simulink model "Open_scen_lucie_test_cs"  (R2019a)
settings: Solver=ode5  StartTime=0.0  StopTime=60  FixedStep=1/60  RelTol=1e-3
PreLoadFcn:
  | mbxruntime.callbacks.PreLoadFcn(bdroot);
PostLoadFcn:
  | mbxruntime.callbacks.PostLoadFcn(bdroot);
InitFcn:
  | mbxruntime.callbacks.InitFcn(bdroot);
StartFcn:
  | mbxruntime.callbacks.StartFcn(bdroot);
StopFcn:
  | mbxruntime.callbacks.StopFcn(bdroot);
model workspace: external: MAT-File .\Open_scen_lucie_test_cs_hws.mat (data not in the file)
undefined symbols (not defined in the file or in its folder): DiscIntNeverNeededParam, FovAzimuth, FovAzimuthDefined, FovElevation, FovElevationDefined, InitImageOutputDir, LocationX, LocationXDefined, LocationY, LocationYDefined, LocationZ, LocationZDefined, mbxruntime, Open_scen_lucie_test_cs_05b3fdca6ec99adc, Open_scen_lucie_test_cs_2d1bc0fbf6141b87, Open_scen_lucie_test_cs_453760b7ad36561d, Open_scen_lucie_test_cs_54de7300b247ce0d, Open_scen_lucie_test_cs_6819f386244a4b71, Open_scen_lucie_test_cs_685351e056f1bd0b, Open_scen_lucie_test_cs_6cd7f038842b0b77, Open_scen_lucie_test_cs_7a35ff65ce771bf6, Open_scen_lucie_test_cs_7ca083c9065fb1a1, Open_scen_lucie_test_cs_8bffacb258fa391b, Open_scen_lucie_test_cs_90e3bd399387ee5e, Open_scen_lucie_test_cs_a1176fb0c2e52fd1, Open_scen_lucie_test_cs_bb93306955583605, Open_scen_lucie_test_cs_c100ca66a180e443, Open_scen_lucie_test_cs_c1ddb1ec4c47a5f8, Open_scen_lucie_test_cs_ee3cfcef3d4d50fa, Open_scen_lucie_test_cs_f0142b471b498fb5, Open_scen_lucie_test_cs_fad1968c5de81336, OrientationPitch, OrientationPitchDefined, OrientationRoll, OrientationRollDefined, OrientationYaw, OrientationYawDefined, tabledata
libraries: adeye_lib x15, PreScanSimulinkLibrary x6, PreScanUsefulBlocks x1, simulink x1
(part 7 of 8)

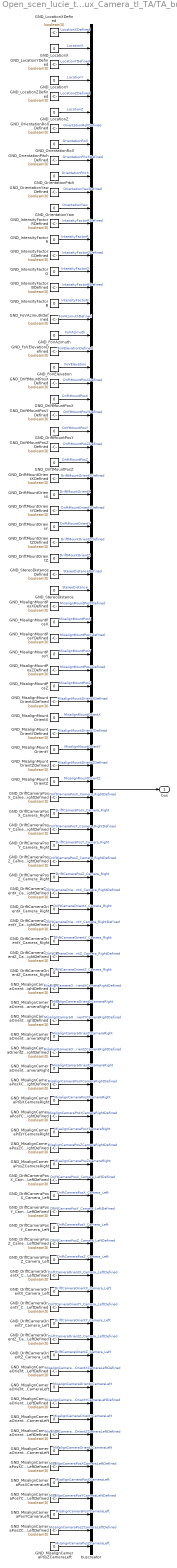
== system Open_scen_lucie_test_cs/BMW_X5_SUV_1/Mux_Camera_tl_TA/TA_bus ==
  GND_DriftCameraOrientX_Camera_Left : Constant  Value=0
  GND_DriftCameraOrientX_Camera_LeftDefined : Constant  Value=boolean(0)
  GND_DriftCameraOrientX_Camera_Right : Constant  Value=0
  GND_DriftCameraOrientX_Camera_RightDefined : Constant  Value=boolean(0)
  GND_DriftCameraOrientY_Camera_Left : Constant  Value=0
  GND_DriftCameraOrientY_Camera_LeftDefined : Constant  Value=boolean(0)
  GND_DriftCameraOrientY_Camera_Right : Constant  Value=0
  GND_DriftCameraOrientY_Camera_RightDefined : Constant  Value=boolean(0)
  GND_DriftCameraOrientZ_Camera_Left : Constant  Value=0
  GND_DriftCameraOrientZ_Camera_LeftDefined : Constant  Value=boolean(0)
  GND_DriftCameraOrientZ_Camera_Right : Constant  Value=0
  GND_DriftCameraOrientZ_Camera_RightDefined : Constant  Value=boolean(0)
  GND_DriftCameraPosX_Camera_Left : Constant  Value=0
  GND_DriftCameraPosX_Camera_LeftDefined : Constant  Value=boolean(0)
  GND_DriftCameraPosX_Camera_Right : Constant  Value=0
  GND_DriftCameraPosX_Camera_RightDefined : Constant  Value=boolean(0)
  GND_DriftCameraPosY_Camera_Left : Constant  Value=0
  GND_DriftCameraPosY_Camera_LeftDefined : Constant  Value=boolean(0)
  GND_DriftCameraPosY_Camera_Right : Constant  Value=0
  GND_DriftCameraPosY_Camera_RightDefined : Constant  Value=boolean(0)
  GND_DriftCameraPosZ_Camera_Left : Constant  Value=0
  GND_DriftCameraPosZ_Camera_LeftDefined : Constant  Value=boolean(0)
  GND_DriftCameraPosZ_Camera_Right : Constant  Value=0
  GND_DriftCameraPosZ_Camera_RightDefined : Constant  Value=boolean(0)
  GND_DriftMountOrientX : Constant  Value=0
  GND_DriftMountOrientXDefined : Constant  Value=boolean(0)
  GND_DriftMountOrientY : Constant  Value=0
  GND_DriftMountOrientYDefined : Constant  Value=boolean(0)
  GND_DriftMountOrientZ : Constant  Value=0
  GND_DriftMountOrientZDefined : Constant  Value=boolean(0)
  GND_DriftMountPosX : Constant  Value=0
  GND_DriftMountPosXDefined : Constant  Value=boolean(0)
  GND_DriftMountPosY : Constant  Value=0
  GND_DriftMountPosYDefined : Constant  Value=boolean(0)
  GND_DriftMountPosZ : Constant  Value=0
  GND_DriftMountPosZDefined : Constant  Value=boolean(0)
  GND_FoVAzimuth : Constant  Value=0
  GND_FoVAzimuthDefined : Constant  Value=boolean(0)
  GND_FoVElevation : Constant  Value=0
  GND_FoVElevationDefined : Constant  Value=boolean(0)
  GND_IntensityFactorB : Constant  Value=0
  GND_IntensityFactorBDefined : Constant  Value=boolean(0)
  GND_IntensityFactorG : Constant  Value=0
  GND_IntensityFactorGDefined : Constant  Value=boolean(0)
  GND_IntensityFactorR : Constant  Value=0
  GND_IntensityFactorRDefined : Constant  Value=boolean(0)
  GND_LocationX : Constant  Value=0
  GND_LocationXDefined : Constant  Value=boolean(0)
  GND_LocationY : Constant  Value=0
  GND_LocationYDefined : Constant  Value=boolean(0)
  GND_LocationZ : Constant  Value=0
  GND_LocationZDefined : Constant  Value=boolean(0)
  GND_MisalignCameraOrientXCameraLeft : Constant  Value=0
  GND_MisalignCameraOrientXCameraLeftDefined : Constant  Value=boolean(0)
  GND_MisalignCameraOrientXCameraRight : Constant  Value=0
  GND_MisalignCameraOrientXCameraRightDefined : Constant  Value=boolean(0)
  GND_MisalignCameraOrientYCameraLeft : Constant  Value=0
  GND_MisalignCameraOrientYCameraLeftDefined : Constant  Value=boolean(0)
  GND_MisalignCameraOrientYCameraRight : Constant  Value=0
  GND_MisalignCameraOrientYCameraRightDefined : Constant  Value=boolean(0)
  GND_MisalignCameraOrientZCameraLeft : Constant  Value=0
  GND_MisalignCameraOrientZCameraLeftDefined : Constant  Value=boolean(0)
  GND_MisalignCameraOrientZCameraRight : Constant  Value=0
  GND_MisalignCameraOrientZCameraRightDefined : Constant  Value=boolean(0)
  GND_MisalignCameraPosXCameraLeft : Constant  Value=0
  GND_MisalignCameraPosXCameraLeftDefined : Constant  Value=boolean(0)
  GND_MisalignCameraPosXCameraRight : Constant  Value=0
  GND_MisalignCameraPosXCameraRightDefined : Constant  Value=boolean(0)
  GND_MisalignCameraPosYCameraLeft : Constant  Value=0
  GND_MisalignCameraPosYCameraLeftDefined : Constant  Value=boolean(0)
  GND_MisalignCameraPosYCameraRight : Constant  Value=0
  GND_MisalignCameraPosYCameraRightDefined : Constant  Value=boolean(0)
  GND_MisalignCameraPosZCameraLeft : Constant  Value=0
  GND_MisalignCameraPosZCameraLeftDefined : Constant  Value=boolean(0)
  GND_MisalignCameraPosZCameraRight : Constant  Value=0
  GND_MisalignCameraPosZCameraRightDefined : Constant  Value=boolean(0)
  GND_MisalignMountOrientX : Constant  Value=0
  GND_MisalignMountOrientXDefined : Constant  Value=boolean(0)
  GND_MisalignMountOrientY : Constant  Value=0
  GND_MisalignMountOrientYDefined : Constant  Value=boolean(0)
  GND_MisalignMountOrientZ : Constant  Value=0
  GND_MisalignMountOrientZDefined : Constant  Value=boolean(0)
  GND_MisalignMountPosX : Constant  Value=0
  GND_MisalignMountPosXDefined : Constant  Value=boolean(0)
  GND_MisalignMountPosY : Constant  Value=0
  GND_MisalignMountPosYDefined : Constant  Value=boolean(0)
  GND_MisalignMountPosZ : Constant  Value=0
  GND_MisalignMountPosZDefined : Constant  Value=boolean(0)
  GND_OrientationPitch : Constant  Value=0
  GND_OrientationPitchDefined : Constant  Value=boolean(0)
  GND_OrientationRoll : Constant  Value=0
  GND_OrientationRollDefined : Constant  Value=boolean(0)
  GND_OrientationYaw : Constant  Value=0
  GND_OrientationYawDefined : Constant  Value=boolean(0)
  GND_StereoDistance : Constant  Value=0
  GND_StereoDistanceDefined : Constant  Value=boolean(0)
  buscreator : BusCreator  Inputs=96  OutDataTypeStr=Bus: PRESCAN_CAMERASENSOR_TA  NonVirtualBus=on
  bus : Outport  OutDataTypeStr=Bus: PRESCAN_CAMERASENSOR_TA
  wires:
  GND_LocationXDefined/1 -> buscreator/1  "LocationXDefined"
  GND_LocationX/1 -> buscreator/2  "LocationX"
  GND_LocationYDefined/1 -> buscreator/3  "LocationYDefined"
  GND_LocationY/1 -> buscreator/4  "LocationY"
  GND_LocationZDefined/1 -> buscreator/5  "LocationZDefined"
  GND_LocationZ/1 -> buscreator/6  "LocationZ"
  GND_OrientationRollDefined/1 -> buscreator/7  "OrientationRollDefined"
  GND_OrientationRoll/1 -> buscreator/8  "OrientationRoll"
  GND_OrientationPitchDefined/1 -> buscreator/9  "OrientationPitchDefined"
  GND_OrientationPitch/1 -> buscreator/10  "OrientationPitch"
  GND_OrientationYawDefined/1 -> buscreator/11  "OrientationYawDefined"
  GND_OrientationYaw/1 -> buscreator/12  "OrientationYaw"
  GND_IntensityFactorRDefined/1 -> buscreator/13  "IntensityFactorRDefined"
  GND_IntensityFactorR/1 -> buscreator/14  "IntensityFactorR"
  GND_IntensityFactorGDefined/1 -> buscreator/15  "IntensityFactorGDefined"
  GND_IntensityFactorG/1 -> buscreator/16  "IntensityFactorG"
  GND_IntensityFactorBDefined/1 -> buscreator/17  "IntensityFactorBDefined"
  GND_IntensityFactorB/1 -> buscreator/18  "IntensityFactorB"
  GND_FoVAzimuthDefined/1 -> buscreator/19  "FoVAzimuthDefined"
  GND_FoVAzimuth/1 -> buscreator/20  "FoVAzimuth"
  GND_FoVElevationDefined/1 -> buscreator/21  "FoVElevationDefined"
  GND_FoVElevation/1 -> buscreator/22  "FoVElevation"
  GND_DriftMountPosXDefined/1 -> buscreator/23  "DriftMountPosXDefined"
  GND_DriftMountPosX/1 -> buscreator/24  "DriftMountPosX"
  GND_DriftMountPosYDefined/1 -> buscreator/25  "DriftMountPosYDefined"
  GND_DriftMountPosY/1 -> buscreator/26  "DriftMountPosY"
  GND_DriftMountPosZDefined/1 -> buscreator/27  "DriftMountPosZDefined"
  GND_DriftMountPosZ/1 -> buscreator/28  "DriftMountPosZ"
  GND_DriftMountOrientXDefined/1 -> buscreator/29  "DriftMountOrientXDefined"
  GND_DriftMountOrientX/1 -> buscreator/30  "DriftMountOrientX"
  GND_DriftMountOrientYDefined/1 -> buscreator/31  "DriftMountOrientYDefined"
  GND_DriftMountOrientY/1 -> buscreator/32  "DriftMountOrientY"
  GND_DriftMountOrientZDefined/1 -> buscreator/33  "DriftMountOrientZDefined"
  GND_DriftMountOrientZ/1 -> buscreator/34  "DriftMountOrientZ"
  GND_StereoDistanceDefined/1 -> buscreator/35  "StereoDistanceDefined"
  GND_StereoDistance/1 -> buscreator/36  "StereoDistance"
  GND_MisalignMountPosXDefined/1 -> buscreator/37  "MisalignMountPosXDefined"
  GND_MisalignMountPosX/1 -> buscreator/38  "MisalignMountPosX"
  GND_MisalignMountPosYDefined/1 -> buscreator/39  "MisalignMountPosYDefined"
  GND_MisalignMountPosY/1 -> buscreator/40  "MisalignMountPosY"
  GND_MisalignMountPosZDefined/1 -> buscreator/41  "MisalignMountPosZDefined"
  GND_MisalignMountPosZ/1 -> buscreator/42  "MisalignMountPosZ"
  GND_MisalignMountOrientXDefined/1 -> buscreator/43  "MisalignMountOrientXDefined"
  GND_MisalignMountOrientX/1 -> buscreator/44  "MisalignMountOrientX"
  GND_MisalignMountOrientYDefined/1 -> buscreator/45  "MisalignMountOrientYDefined"
  GND_MisalignMountOrientY/1 -> buscreator/46  "MisalignMountOrientY"
  GND_MisalignMountOrientZDefined/1 -> buscreator/47  "MisalignMountOrientZDefined"
  GND_MisalignMountOrientZ/1 -> buscreator/48  "MisalignMountOrientZ"
  GND_DriftCameraPosX_Camera_RightDefined/1 -> buscreator/49  "DriftCameraPosX_Camera_RightDefined"
  GND_DriftCameraPosX_Camera_Right/1 -> buscreator/50  "DriftCameraPosX_Camera_Right"
  GND_DriftCameraPosY_Camera_RightDefined/1 -> buscreator/51  "DriftCameraPosY_Camera_RightDefined"
  GND_DriftCameraPosY_Camera_Right/1 -> buscreator/52  "DriftCameraPosY_Camera_Right"
  GND_DriftCameraPosZ_Camera_RightDefined/1 -> buscreator/53  "DriftCameraPosZ_Camera_RightDefined"
  GND_DriftCameraPosZ_Camera_Right/1 -> buscreator/54  "DriftCameraPosZ_Camera_Right"
  GND_DriftCameraOrientX_Camera_RightDefined/1 -> buscreator/55  "DriftCameraOrientX_Camera_RightDefined"
  GND_DriftCameraOrientX_Camera_Right/1 -> buscreator/56  "DriftCameraOrientX_Camera_Right"
  GND_DriftCameraOrientY_Camera_RightDefined/1 -> buscreator/57  "DriftCameraOrientY_Camera_RightDefined"
  GND_DriftCameraOrientY_Camera_Right/1 -> buscreator/58  "DriftCameraOrientY_Camera_Right"
  GND_DriftCameraOrientZ_Camera_RightDefined/1 -> buscreator/59  "DriftCameraOrientZ_Camera_RightDefined"
  GND_DriftCameraOrientZ_Camera_Right/1 -> buscreator/60  "DriftCameraOrientZ_Camera_Right"
  GND_MisalignCameraOrientXCameraRightDefined/1 -> buscreator/61  "MisalignCameraOrientXCameraRightDefined"
  GND_MisalignCameraOrientXCameraRight/1 -> buscreator/62  "MisalignCameraOrientXCameraRight"
  GND_MisalignCameraOrientYCameraRightDefined/1 -> buscreator/63  "MisalignCameraOrientYCameraRightDefined"
  GND_MisalignCameraOrientYCameraRight/1 -> buscreator/64  "MisalignCameraOrientYCameraRight"
  GND_MisalignCameraOrientZCameraRightDefined/1 -> buscreator/65  "MisalignCameraOrientZCameraRightDefined"
  GND_MisalignCameraOrientZCameraRight/1 -> buscreator/66  "MisalignCameraOrientZCameraRight"
  GND_MisalignCameraPosXCameraRightDefined/1 -> buscreator/67  "MisalignCameraPosXCameraRightDefined"
  GND_MisalignCameraPosXCameraRight/1 -> buscreator/68  "MisalignCameraPosXCameraRight"
  GND_MisalignCameraPosYCameraRightDefined/1 -> buscreator/69  "MisalignCameraPosYCameraRightDefined"
  GND_MisalignCameraPosYCameraRight/1 -> buscreator/70  "MisalignCameraPosYCameraRight"
  GND_MisalignCameraPosZCameraRightDefined/1 -> buscreator/71  "MisalignCameraPosZCameraRightDefined"
  GND_MisalignCameraPosZCameraRight/1 -> buscreator/72  "MisalignCameraPosZCameraRight"
  GND_DriftCameraPosX_Camera_LeftDefined/1 -> buscreator/73  "DriftCameraPosX_Camera_LeftDefined"
  GND_DriftCameraPosX_Camera_Left/1 -> buscreator/74  "DriftCameraPosX_Camera_Left"
  GND_DriftCameraPosY_Camera_LeftDefined/1 -> buscreator/75  "DriftCameraPosY_Camera_LeftDefined"
  GND_DriftCameraPosY_Camera_Left/1 -> buscreator/76  "DriftCameraPosY_Camera_Left"
  GND_DriftCameraPosZ_Camera_LeftDefined/1 -> buscreator/77  "DriftCameraPosZ_Camera_LeftDefined"
  GND_DriftCameraPosZ_Camera_Left/1 -> buscreator/78  "DriftCameraPosZ_Camera_Left"
  GND_DriftCameraOrientX_Camera_LeftDefined/1 -> buscreator/79  "DriftCameraOrientX_Camera_LeftDefined"
  GND_DriftCameraOrientX_Camera_Left/1 -> buscreator/80  "DriftCameraOrientX_Camera_Left"
  GND_DriftCameraOrientY_Camera_LeftDefined/1 -> buscreator/81  "DriftCameraOrientY_Camera_LeftDefined"
  GND_DriftCameraOrientY_Camera_Left/1 -> buscreator/82  "DriftCameraOrientY_Camera_Left"
  GND_DriftCameraOrientZ_Camera_LeftDefined/1 -> buscreator/83  "DriftCameraOrientZ_Camera_LeftDefined"
  GND_DriftCameraOrientZ_Camera_Left/1 -> buscreator/84  "DriftCameraOrientZ_Camera_Left"
  GND_MisalignCameraOrientXCameraLeftDefined/1 -> buscreator/85  "MisalignCameraOrientXCameraLeftDefined"
  GND_MisalignCameraOrientXCameraLeft/1 -> buscreator/86  "MisalignCameraOrientXCameraLeft"
  GND_MisalignCameraOrientYCameraLeftDefined/1 -> buscreator/87  "MisalignCameraOrientYCameraLeftDefined"
  GND_MisalignCameraOrientYCameraLeft/1 -> buscreator/88  "MisalignCameraOrientYCameraLeft"
  GND_MisalignCameraOrientZCameraLeftDefined/1 -> buscreator/89  "MisalignCameraOrientZCameraLeftDefined"
  GND_MisalignCameraOrientZCameraLeft/1 -> buscreator/90  "MisalignCameraOrientZCameraLeft"
  GND_MisalignCameraPosXCameraLeftDefined/1 -> buscreator/91  "MisalignCameraPosXCameraLeftDefined"
  GND_MisalignCameraPosXCameraLeft/1 -> buscreator/92  "MisalignCameraPosXCameraLeft"
  GND_MisalignCameraPosYCameraLeftDefined/1 -> buscreator/93  "MisalignCameraPosYCameraLeftDefined"
  GND_MisalignCameraPosYCameraLeft/1 -> buscreator/94  "MisalignCameraPosYCameraLeft"
  GND_MisalignCameraPosZCameraLeftDefined/1 -> buscreator/95  "MisalignCameraPosZCameraLeftDefined"
  GND_MisalignCameraPosZCameraLeft/1 -> buscreator/96  "MisalignCameraPosZCameraLeft"
  buscreator/1 -> bus/1

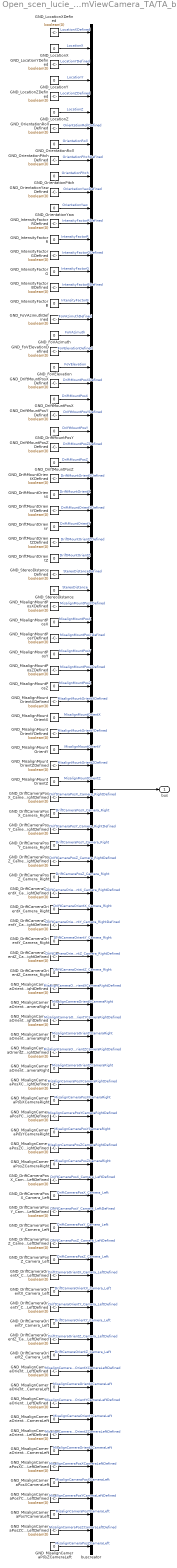
== system Open_scen_lucie_test_cs/BMW_X5_SUV_1/Mux_HumViewCamera_TA/TA_bus ==
  GND_DriftCameraOrientX_Camera_Left : Constant  Value=0
  GND_DriftCameraOrientX_Camera_LeftDefined : Constant  Value=boolean(0)
  GND_DriftCameraOrientX_Camera_Right : Constant  Value=0
  GND_DriftCameraOrientX_Camera_RightDefined : Constant  Value=boolean(0)
  GND_DriftCameraOrientY_Camera_Left : Constant  Value=0
  GND_DriftCameraOrientY_Camera_LeftDefined : Constant  Value=boolean(0)
  GND_DriftCameraOrientY_Camera_Right : Constant  Value=0
  GND_DriftCameraOrientY_Camera_RightDefined : Constant  Value=boolean(0)
  GND_DriftCameraOrientZ_Camera_Left : Constant  Value=0
  GND_DriftCameraOrientZ_Camera_LeftDefined : Constant  Value=boolean(0)
  GND_DriftCameraOrientZ_Camera_Right : Constant  Value=0
  GND_DriftCameraOrientZ_Camera_RightDefined : Constant  Value=boolean(0)
  GND_DriftCameraPosX_Camera_Left : Constant  Value=0
  GND_DriftCameraPosX_Camera_LeftDefined : Constant  Value=boolean(0)
  GND_DriftCameraPosX_Camera_Right : Constant  Value=0
  GND_DriftCameraPosX_Camera_RightDefined : Constant  Value=boolean(0)
  GND_DriftCameraPosY_Camera_Left : Constant  Value=0
  GND_DriftCameraPosY_Camera_LeftDefined : Constant  Value=boolean(0)
  GND_DriftCameraPosY_Camera_Right : Constant  Value=0
  GND_DriftCameraPosY_Camera_RightDefined : Constant  Value=boolean(0)
  GND_DriftCameraPosZ_Camera_Left : Constant  Value=0
  GND_DriftCameraPosZ_Camera_LeftDefined : Constant  Value=boolean(0)
  GND_DriftCameraPosZ_Camera_Right : Constant  Value=0
  GND_DriftCameraPosZ_Camera_RightDefined : Constant  Value=boolean(0)
  GND_DriftMountOrientX : Constant  Value=0
  GND_DriftMountOrientXDefined : Constant  Value=boolean(0)
  GND_DriftMountOrientY : Constant  Value=0
  GND_DriftMountOrientYDefined : Constant  Value=boolean(0)
  GND_DriftMountOrientZ : Constant  Value=0
  GND_DriftMountOrientZDefined : Constant  Value=boolean(0)
  GND_DriftMountPosX : Constant  Value=0
  GND_DriftMountPosXDefined : Constant  Value=boolean(0)
  GND_DriftMountPosY : Constant  Value=0
  GND_DriftMountPosYDefined : Constant  Value=boolean(0)
  GND_DriftMountPosZ : Constant  Value=0
  GND_DriftMountPosZDefined : Constant  Value=boolean(0)
  GND_FoVAzimuth : Constant  Value=0
  GND_FoVAzimuthDefined : Constant  Value=boolean(0)
  GND_FoVElevation : Constant  Value=0
  GND_FoVElevationDefined : Constant  Value=boolean(0)
  GND_IntensityFactorB : Constant  Value=0
  GND_IntensityFactorBDefined : Constant  Value=boolean(0)
  GND_IntensityFactorG : Constant  Value=0
  GND_IntensityFactorGDefined : Constant  Value=boolean(0)
  GND_IntensityFactorR : Constant  Value=0
  GND_IntensityFactorRDefined : Constant  Value=boolean(0)
  GND_LocationX : Constant  Value=0
  GND_LocationXDefined : Constant  Value=boolean(0)
  GND_LocationY : Constant  Value=0
  GND_LocationYDefined : Constant  Value=boolean(0)
  GND_LocationZ : Constant  Value=0
  GND_LocationZDefined : Constant  Value=boolean(0)
  GND_MisalignCameraOrientXCameraLeft : Constant  Value=0
  GND_MisalignCameraOrientXCameraLeftDefined : Constant  Value=boolean(0)
  GND_MisalignCameraOrientXCameraRight : Constant  Value=0
  GND_MisalignCameraOrientXCameraRightDefined : Constant  Value=boolean(0)
  GND_MisalignCameraOrientYCameraLeft : Constant  Value=0
  GND_MisalignCameraOrientYCameraLeftDefined : Constant  Value=boolean(0)
  GND_MisalignCameraOrientYCameraRight : Constant  Value=0
  GND_MisalignCameraOrientYCameraRightDefined : Constant  Value=boolean(0)
  GND_MisalignCameraOrientZCameraLeft : Constant  Value=0
  GND_MisalignCameraOrientZCameraLeftDefined : Constant  Value=boolean(0)
  GND_MisalignCameraOrientZCameraRight : Constant  Value=0
  GND_MisalignCameraOrientZCameraRightDefined : Constant  Value=boolean(0)
  GND_MisalignCameraPosXCameraLeft : Constant  Value=0
  GND_MisalignCameraPosXCameraLeftDefined : Constant  Value=boolean(0)
  GND_MisalignCameraPosXCameraRight : Constant  Value=0
  GND_MisalignCameraPosXCameraRightDefined : Constant  Value=boolean(0)
  GND_MisalignCameraPosYCameraLeft : Constant  Value=0
  GND_MisalignCameraPosYCameraLeftDefined : Constant  Value=boolean(0)
  GND_MisalignCameraPosYCameraRight : Constant  Value=0
  GND_MisalignCameraPosYCameraRightDefined : Constant  Value=boolean(0)
  GND_MisalignCameraPosZCameraLeft : Constant  Value=0
  GND_MisalignCameraPosZCameraLeftDefined : Constant  Value=boolean(0)
  GND_MisalignCameraPosZCameraRight : Constant  Value=0
  GND_MisalignCameraPosZCameraRightDefined : Constant  Value=boolean(0)
  GND_MisalignMountOrientX : Constant  Value=0
  GND_MisalignMountOrientXDefined : Constant  Value=boolean(0)
  GND_MisalignMountOrientY : Constant  Value=0
  GND_MisalignMountOrientYDefined : Constant  Value=boolean(0)
  GND_MisalignMountOrientZ : Constant  Value=0
  GND_MisalignMountOrientZDefined : Constant  Value=boolean(0)
  GND_MisalignMountPosX : Constant  Value=0
  GND_MisalignMountPosXDefined : Constant  Value=boolean(0)
  GND_MisalignMountPosY : Constant  Value=0
  GND_MisalignMountPosYDefined : Constant  Value=boolean(0)
  GND_MisalignMountPosZ : Constant  Value=0
  GND_MisalignMountPosZDefined : Constant  Value=boolean(0)
  GND_OrientationPitch : Constant  Value=0
  GND_OrientationPitchDefined : Constant  Value=boolean(0)
  GND_OrientationRoll : Constant  Value=0
  GND_OrientationRollDefined : Constant  Value=boolean(0)
  GND_OrientationYaw : Constant  Value=0
  GND_OrientationYawDefined : Constant  Value=boolean(0)
  GND_StereoDistance : Constant  Value=0
  GND_StereoDistanceDefined : Constant  Value=boolean(0)
  buscreator : BusCreator  Inputs=96  OutDataTypeStr=Bus: PRESCAN_CAMERASENSOR_TA  NonVirtualBus=on
  bus : Outport  OutDataTypeStr=Bus: PRESCAN_CAMERASENSOR_TA
  wires:
  GND_LocationXDefined/1 -> buscreator/1  "LocationXDefined"
  GND_LocationX/1 -> buscreator/2  "LocationX"
  GND_LocationYDefined/1 -> buscreator/3  "LocationYDefined"
  GND_LocationY/1 -> buscreator/4  "LocationY"
  GND_LocationZDefined/1 -> buscreator/5  "LocationZDefined"
  GND_LocationZ/1 -> buscreator/6  "LocationZ"
  GND_OrientationRollDefined/1 -> buscreator/7  "OrientationRollDefined"
  GND_OrientationRoll/1 -> buscreator/8  "OrientationRoll"
  GND_OrientationPitchDefined/1 -> buscreator/9  "OrientationPitchDefined"
  GND_OrientationPitch/1 -> buscreator/10  "OrientationPitch"
  GND_OrientationYawDefined/1 -> buscreator/11  "OrientationYawDefined"
  GND_OrientationYaw/1 -> buscreator/12  "OrientationYaw"
  GND_IntensityFactorRDefined/1 -> buscreator/13  "IntensityFactorRDefined"
  GND_IntensityFactorR/1 -> buscreator/14  "IntensityFactorR"
  GND_IntensityFactorGDefined/1 -> buscreator/15  "IntensityFactorGDefined"
  GND_IntensityFactorG/1 -> buscreator/16  "IntensityFactorG"
  GND_IntensityFactorBDefined/1 -> buscreator/17  "IntensityFactorBDefined"
  GND_IntensityFactorB/1 -> buscreator/18  "IntensityFactorB"
  GND_FoVAzimuthDefined/1 -> buscreator/19  "FoVAzimuthDefined"
  GND_FoVAzimuth/1 -> buscreator/20  "FoVAzimuth"
  GND_FoVElevationDefined/1 -> buscreator/21  "FoVElevationDefined"
  GND_FoVElevation/1 -> buscreator/22  "FoVElevation"
  GND_DriftMountPosXDefined/1 -> buscreator/23  "DriftMountPosXDefined"
  GND_DriftMountPosX/1 -> buscreator/24  "DriftMountPosX"
  GND_DriftMountPosYDefined/1 -> buscreator/25  "DriftMountPosYDefined"
  GND_DriftMountPosY/1 -> buscreator/26  "DriftMountPosY"
  GND_DriftMountPosZDefined/1 -> buscreator/27  "DriftMountPosZDefined"
  GND_DriftMountPosZ/1 -> buscreator/28  "DriftMountPosZ"
  GND_DriftMountOrientXDefined/1 -> buscreator/29  "DriftMountOrientXDefined"
  GND_DriftMountOrientX/1 -> buscreator/30  "DriftMountOrientX"
  GND_DriftMountOrientYDefined/1 -> buscreator/31  "DriftMountOrientYDefined"
  GND_DriftMountOrientY/1 -> buscreator/32  "DriftMountOrientY"
  GND_DriftMountOrientZDefined/1 -> buscreator/33  "DriftMountOrientZDefined"
  GND_DriftMountOrientZ/1 -> buscreator/34  "DriftMountOrientZ"
  GND_StereoDistanceDefined/1 -> buscreator/35  "StereoDistanceDefined"
  GND_StereoDistance/1 -> buscreator/36  "StereoDistance"
  GND_MisalignMountPosXDefined/1 -> buscreator/37  "MisalignMountPosXDefined"
  GND_MisalignMountPosX/1 -> buscreator/38  "MisalignMountPosX"
  GND_MisalignMountPosYDefined/1 -> buscreator/39  "MisalignMountPosYDefined"
  GND_MisalignMountPosY/1 -> buscreator/40  "MisalignMountPosY"
  GND_MisalignMountPosZDefined/1 -> buscreator/41  "MisalignMountPosZDefined"
  GND_MisalignMountPosZ/1 -> buscreator/42  "MisalignMountPosZ"
  GND_MisalignMountOrientXDefined/1 -> buscreator/43  "MisalignMountOrientXDefined"
  GND_MisalignMountOrientX/1 -> buscreator/44  "MisalignMountOrientX"
  GND_MisalignMountOrientYDefined/1 -> buscreator/45  "MisalignMountOrientYDefined"
  GND_MisalignMountOrientY/1 -> buscreator/46  "MisalignMountOrientY"
  GND_MisalignMountOrientZDefined/1 -> buscreator/47  "MisalignMountOrientZDefined"
  GND_MisalignMountOrientZ/1 -> buscreator/48  "MisalignMountOrientZ"
  GND_DriftCameraPosX_Camera_RightDefined/1 -> buscreator/49  "DriftCameraPosX_Camera_RightDefined"
  GND_DriftCameraPosX_Camera_Right/1 -> buscreator/50  "DriftCameraPosX_Camera_Right"
  GND_DriftCameraPosY_Camera_RightDefined/1 -> buscreator/51  "DriftCameraPosY_Camera_RightDefined"
  GND_DriftCameraPosY_Camera_Right/1 -> buscreator/52  "DriftCameraPosY_Camera_Right"
  GND_DriftCameraPosZ_Camera_RightDefined/1 -> buscreator/53  "DriftCameraPosZ_Camera_RightDefined"
  GND_DriftCameraPosZ_Camera_Right/1 -> buscreator/54  "DriftCameraPosZ_Camera_Right"
  GND_DriftCameraOrientX_Camera_RightDefined/1 -> buscreator/55  "DriftCameraOrientX_Camera_RightDefined"
  GND_DriftCameraOrientX_Camera_Right/1 -> buscreator/56  "DriftCameraOrientX_Camera_Right"
  GND_DriftCameraOrientY_Camera_RightDefined/1 -> buscreator/57  "DriftCameraOrientY_Camera_RightDefined"
  GND_DriftCameraOrientY_Camera_Right/1 -> buscreator/58  "DriftCameraOrientY_Camera_Right"
  GND_DriftCameraOrientZ_Camera_RightDefined/1 -> buscreator/59  "DriftCameraOrientZ_Camera_RightDefined"
  GND_DriftCameraOrientZ_Camera_Right/1 -> buscreator/60  "DriftCameraOrientZ_Camera_Right"
  GND_MisalignCameraOrientXCameraRightDefined/1 -> buscreator/61  "MisalignCameraOrientXCameraRightDefined"
  GND_MisalignCameraOrientXCameraRight/1 -> buscreator/62  "MisalignCameraOrientXCameraRight"
  GND_MisalignCameraOrientYCameraRightDefined/1 -> buscreator/63  "MisalignCameraOrientYCameraRightDefined"
  GND_MisalignCameraOrientYCameraRight/1 -> buscreator/64  "MisalignCameraOrientYCameraRight"
  GND_MisalignCameraOrientZCameraRightDefined/1 -> buscreator/65  "MisalignCameraOrientZCameraRightDefined"
  GND_MisalignCameraOrientZCameraRight/1 -> buscreator/66  "MisalignCameraOrientZCameraRight"
  GND_MisalignCameraPosXCameraRightDefined/1 -> buscreator/67  "MisalignCameraPosXCameraRightDefined"
  GND_MisalignCameraPosXCameraRight/1 -> buscreator/68  "MisalignCameraPosXCameraRight"
  GND_MisalignCameraPosYCameraRightDefined/1 -> buscreator/69  "MisalignCameraPosYCameraRightDefined"
  GND_MisalignCameraPosYCameraRight/1 -> buscreator/70  "MisalignCameraPosYCameraRight"
  GND_MisalignCameraPosZCameraRightDefined/1 -> buscreator/71  "MisalignCameraPosZCameraRightDefined"
  GND_MisalignCameraPosZCameraRight/1 -> buscreator/72  "MisalignCameraPosZCameraRight"
  GND_DriftCameraPosX_Camera_LeftDefined/1 -> buscreator/73  "DriftCameraPosX_Camera_LeftDefined"
  GND_DriftCameraPosX_Camera_Left/1 -> buscreator/74  "DriftCameraPosX_Camera_Left"
  GND_DriftCameraPosY_Camera_LeftDefined/1 -> buscreator/75  "DriftCameraPosY_Camera_LeftDefined"
  GND_DriftCameraPosY_Camera_Left/1 -> buscreator/76  "DriftCameraPosY_Camera_Left"
  GND_DriftCameraPosZ_Camera_LeftDefined/1 -> buscreator/77  "DriftCameraPosZ_Camera_LeftDefined"
  GND_DriftCameraPosZ_Camera_Left/1 -> buscreator/78  "DriftCameraPosZ_Camera_Left"
  GND_DriftCameraOrientX_Camera_LeftDefined/1 -> buscreator/79  "DriftCameraOrientX_Camera_LeftDefined"
  GND_DriftCameraOrientX_Camera_Left/1 -> buscreator/80  "DriftCameraOrientX_Camera_Left"
  GND_DriftCameraOrientY_Camera_LeftDefined/1 -> buscreator/81  "DriftCameraOrientY_Camera_LeftDefined"
  GND_DriftCameraOrientY_Camera_Left/1 -> buscreator/82  "DriftCameraOrientY_Camera_Left"
  GND_DriftCameraOrientZ_Camera_LeftDefined/1 -> buscreator/83  "DriftCameraOrientZ_Camera_LeftDefined"
  GND_DriftCameraOrientZ_Camera_Left/1 -> buscreator/84  "DriftCameraOrientZ_Camera_Left"
  GND_MisalignCameraOrientXCameraLeftDefined/1 -> buscreator/85  "MisalignCameraOrientXCameraLeftDefined"
  GND_MisalignCameraOrientXCameraLeft/1 -> buscreator/86  "MisalignCameraOrientXCameraLeft"
  GND_MisalignCameraOrientYCameraLeftDefined/1 -> buscreator/87  "MisalignCameraOrientYCameraLeftDefined"
  GND_MisalignCameraOrientYCameraLeft/1 -> buscreator/88  "MisalignCameraOrientYCameraLeft"
  GND_MisalignCameraOrientZCameraLeftDefined/1 -> buscreator/89  "MisalignCameraOrientZCameraLeftDefined"
  GND_MisalignCameraOrientZCameraLeft/1 -> buscreator/90  "MisalignCameraOrientZCameraLeft"
  GND_MisalignCameraPosXCameraLeftDefined/1 -> buscreator/91  "MisalignCameraPosXCameraLeftDefined"
  GND_MisalignCameraPosXCameraLeft/1 -> buscreator/92  "MisalignCameraPosXCameraLeft"
  GND_MisalignCameraPosYCameraLeftDefined/1 -> buscreator/93  "MisalignCameraPosYCameraLeftDefined"
  GND_MisalignCameraPosYCameraLeft/1 -> buscreator/94  "MisalignCameraPosYCameraLeft"
  GND_MisalignCameraPosZCameraLeftDefined/1 -> buscreator/95  "MisalignCameraPosZCameraLeftDefined"
  GND_MisalignCameraPosZCameraLeft/1 -> buscreator/96  "MisalignCameraPosZCameraLeft"
  buscreator/1 -> bus/1

== system Open_scen_lucie_test_cs/BMW_X5_SUV_1/Mux_PointCloudSensor_1_TA/TA_bus ==
  GND_FarClippingDistance : Constant  Value=0
  GND_FarClippingDistanceDefined : Constant  Value=boolean(0)
  GND_FovAzimuth : Constant  Value=0
  GND_FovAzimuthDefined : Constant  Value=boolean(0)
  GND_FovElevation : Constant  Value=0
  GND_FovElevationDefined : Constant  Value=boolean(0)
  GND_LocationX : Constant  Value=0
  GND_LocationXDefined : Constant  Value=boolean(0)
  GND_LocationY : Constant  Value=0
  GND_LocationYDefined : Constant  Value=boolean(0)
  GND_LocationZ : Constant  Value=0
  GND_LocationZDefined : Constant  Value=boolean(0)
  GND_NearClippingDistance : Constant  Value=0
  GND_NearClippingDistanceDefined : Constant  Value=boolean(0)
  GND_OrientationPitch : Constant  Value=0
  GND_OrientationPitchDefined : Constant  Value=boolean(0)
  GND_OrientationRoll : Constant  Value=0
  GND_OrientationRollDefined : Constant  Value=boolean(0)
  GND_OrientationYaw : Constant  Value=0
  GND_OrientationYawDefined : Constant  Value=boolean(0)
  buscreator : BusCreator  Inputs=20  OutDataTypeStr=Bus: PRESCAN_PCS_TA_DATA  NonVirtualBus=on
  bus : Outport  OutDataTypeStr=Bus: PRESCAN_PCS_TA_DATA
  wires:
  GND_LocationXDefined/1 -> buscreator/1  "LocationXDefined"
  GND_LocationX/1 -> buscreator/2  "LocationX"
  GND_LocationYDefined/1 -> buscreator/3  "LocationYDefined"
  GND_LocationY/1 -> buscreator/4  "LocationY"
  GND_LocationZDefined/1 -> buscreator/5  "LocationZDefined"
  GND_LocationZ/1 -> buscreator/6  "LocationZ"
  GND_OrientationRollDefined/1 -> buscreator/7  "OrientationRollDefined"
  GND_OrientationRoll/1 -> buscreator/8  "OrientationRoll"
  GND_OrientationPitchDefined/1 -> buscreator/9  "OrientationPitchDefined"
  GND_OrientationPitch/1 -> buscreator/10  "OrientationPitch"
  GND_OrientationYawDefined/1 -> buscreator/11  "OrientationYawDefined"
  GND_OrientationYaw/1 -> buscreator/12  "OrientationYaw"
  GND_FovAzimuthDefined/1 -> buscreator/13  "FovAzimuthDefined"
  GND_FovAzimuth/1 -> buscreator/14  "FovAzimuth"
  GND_FovElevationDefined/1 -> buscreator/15  "FovElevationDefined"
  GND_FovElevation/1 -> buscreator/16  "FovElevation"
  GND_NearClippingDistanceDefined/1 -> buscreator/17  "NearClippingDistanceDefined"
  GND_NearClippingDistance/1 -> buscreator/18  "NearClippingDistance"
  GND_FarClippingDistanceDefined/1 -> buscreator/19  "FarClippingDistanceDefined"
  GND_FarClippingDistance/1 -> buscreator/20  "FarClippingDistance"
  buscreator/1 -> bus/1

== system Open_scen_lucie_test_cs/BMW_X5_SUV_1/Mux_PointCloudSensor_2_TA/TA_bus ==
  GND_FarClippingDistance : Constant  Value=0
  GND_FarClippingDistanceDefined : Constant  Value=boolean(0)
  GND_FovAzimuth : Constant  Value=0
  GND_FovAzimuthDefined : Constant  Value=boolean(0)
  GND_FovElevation : Constant  Value=0
  GND_FovElevationDefined : Constant  Value=boolean(0)
  GND_LocationX : Constant  Value=0
  GND_LocationXDefined : Constant  Value=boolean(0)
  GND_LocationY : Constant  Value=0
  GND_LocationYDefined : Constant  Value=boolean(0)
  GND_LocationZ : Constant  Value=0
  GND_LocationZDefined : Constant  Value=boolean(0)
  GND_NearClippingDistance : Constant  Value=0
  GND_NearClippingDistanceDefined : Constant  Value=boolean(0)
  GND_OrientationPitch : Constant  Value=0
  GND_OrientationPitchDefined : Constant  Value=boolean(0)
  GND_OrientationRoll : Constant  Value=0
  GND_OrientationRollDefined : Constant  Value=boolean(0)
  GND_OrientationYaw : Constant  Value=0
  GND_OrientationYawDefined : Constant  Value=boolean(0)
  buscreator : BusCreator  Inputs=20  OutDataTypeStr=Bus: PRESCAN_PCS_TA_DATA  NonVirtualBus=on
  bus : Outport  OutDataTypeStr=Bus: PRESCAN_PCS_TA_DATA
  wires:
  GND_LocationXDefined/1 -> buscreator/1  "LocationXDefined"
  GND_LocationX/1 -> buscreator/2  "LocationX"
  GND_LocationYDefined/1 -> buscreator/3  "LocationYDefined"
  GND_LocationY/1 -> buscreator/4  "LocationY"
  GND_LocationZDefined/1 -> buscreator/5  "LocationZDefined"
  GND_LocationZ/1 -> buscreator/6  "LocationZ"
  GND_OrientationRollDefined/1 -> buscreator/7  "OrientationRollDefined"
  GND_OrientationRoll/1 -> buscreator/8  "OrientationRoll"
  GND_OrientationPitchDefined/1 -> buscreator/9  "OrientationPitchDefined"
  GND_OrientationPitch/1 -> buscreator/10  "OrientationPitch"
  GND_OrientationYawDefined/1 -> buscreator/11  "OrientationYawDefined"
  GND_OrientationYaw/1 -> buscreator/12  "OrientationYaw"
  GND_FovAzimuthDefined/1 -> buscreator/13  "FovAzimuthDefined"
  GND_FovAzimuth/1 -> buscreator/14  "FovAzimuth"
  GND_FovElevationDefined/1 -> buscreator/15  "FovElevationDefined"
  GND_FovElevation/1 -> buscreator/16  "FovElevation"
  GND_NearClippingDistanceDefined/1 -> buscreator/17  "NearClippingDistanceDefined"
  GND_NearClippingDistance/1 -> buscreator/18  "NearClippingDistance"
  GND_FarClippingDistanceDefined/1 -> buscreator/19  "FarClippingDistanceDefined"
  GND_FarClippingDistance/1 -> buscreator/20  "FarClippingDistance"
  buscreator/1 -> bus/1

== system Open_scen_lucie_test_cs/BMW_X5_SUV_1/Mux_PointCloudSensor_3_TA/TA_bus ==
  GND_FarClippingDistance : Constant  Value=0
  GND_FarClippingDistanceDefined : Constant  Value=boolean(0)
  GND_FovAzimuth : Constant  Value=0
  GND_FovAzimuthDefined : Constant  Value=boolean(0)
  GND_FovElevation : Constant  Value=0
  GND_FovElevationDefined : Constant  Value=boolean(0)
  GND_LocationX : Constant  Value=0
  GND_LocationXDefined : Constant  Value=boolean(0)
  GND_LocationY : Constant  Value=0
  GND_LocationYDefined : Constant  Value=boolean(0)
  GND_LocationZ : Constant  Value=0
  GND_LocationZDefined : Constant  Value=boolean(0)
  GND_NearClippingDistance : Constant  Value=0
  GND_NearClippingDistanceDefined : Constant  Value=boolean(0)
  GND_OrientationPitch : Constant  Value=0
  GND_OrientationPitchDefined : Constant  Value=boolean(0)
  GND_OrientationRoll : Constant  Value=0
  GND_OrientationRollDefined : Constant  Value=boolean(0)
  GND_OrientationYaw : Constant  Value=0
  GND_OrientationYawDefined : Constant  Value=boolean(0)
  buscreator : BusCreator  Inputs=20  OutDataTypeStr=Bus: PRESCAN_PCS_TA_DATA  NonVirtualBus=on
  bus : Outport  OutDataTypeStr=Bus: PRESCAN_PCS_TA_DATA
  wires:
  GND_LocationXDefined/1 -> buscreator/1  "LocationXDefined"
  GND_LocationX/1 -> buscreator/2  "LocationX"
  GND_LocationYDefined/1 -> buscreator/3  "LocationYDefined"
  GND_LocationY/1 -> buscreator/4  "LocationY"
  GND_LocationZDefined/1 -> buscreator/5  "LocationZDefined"
  GND_LocationZ/1 -> buscreator/6  "LocationZ"
  GND_OrientationRollDefined/1 -> buscreator/7  "OrientationRollDefined"
  GND_OrientationRoll/1 -> buscreator/8  "OrientationRoll"
  GND_OrientationPitchDefined/1 -> buscreator/9  "OrientationPitchDefined"
  GND_OrientationPitch/1 -> buscreator/10  "OrientationPitch"
  GND_OrientationYawDefined/1 -> buscreator/11  "OrientationYawDefined"
  GND_OrientationYaw/1 -> buscreator/12  "OrientationYaw"
  GND_FovAzimuthDefined/1 -> buscreator/13  "FovAzimuthDefined"
  GND_FovAzimuth/1 -> buscreator/14  "FovAzimuth"
  GND_FovElevationDefined/1 -> buscreator/15  "FovElevationDefined"
  GND_FovElevation/1 -> buscreator/16  "FovElevation"
  GND_NearClippingDistanceDefined/1 -> buscreator/17  "NearClippingDistanceDefined"
  GND_NearClippingDistance/1 -> buscreator/18  "NearClippingDistance"
  GND_FarClippingDistanceDefined/1 -> buscreator/19  "FarClippingDistanceDefined"
  GND_FarClippingDistance/1 -> buscreator/20  "FarClippingDistance"
  buscreator/1 -> bus/1

== system Open_scen_lucie_test_cs/BMW_X5_SUV_1/Mux_PointCloudSensor_4_TA/TA_bus ==
  GND_FarClippingDistance : Constant  Value=0
  GND_FarClippingDistanceDefined : Constant  Value=boolean(0)
  GND_FovAzimuth : Constant  Value=0
  GND_FovAzimuthDefined : Constant  Value=boolean(0)
  GND_FovElevation : Constant  Value=0
  GND_FovElevationDefined : Constant  Value=boolean(0)
  GND_LocationX : Constant  Value=0
  GND_LocationXDefined : Constant  Value=boolean(0)
  GND_LocationY : Constant  Value=0
  GND_LocationYDefined : Constant  Value=boolean(0)
  GND_LocationZ : Constant  Value=0
  GND_LocationZDefined : Constant  Value=boolean(0)
  GND_NearClippingDistance : Constant  Value=0
  GND_NearClippingDistanceDefined : Constant  Value=boolean(0)
  GND_OrientationPitch : Constant  Value=0
  GND_OrientationPitchDefined : Constant  Value=boolean(0)
  GND_OrientationRoll : Constant  Value=0
  GND_OrientationRollDefined : Constant  Value=boolean(0)
  GND_OrientationYaw : Constant  Value=0
  GND_OrientationYawDefined : Constant  Value=boolean(0)
  buscreator : BusCreator  Inputs=20  OutDataTypeStr=Bus: PRESCAN_PCS_TA_DATA  NonVirtualBus=on
  bus : Outport  OutDataTypeStr=Bus: PRESCAN_PCS_TA_DATA
  wires:
  GND_LocationXDefined/1 -> buscreator/1  "LocationXDefined"
  GND_LocationX/1 -> buscreator/2  "LocationX"
  GND_LocationYDefined/1 -> buscreator/3  "LocationYDefined"
  GND_LocationY/1 -> buscreator/4  "LocationY"
  GND_LocationZDefined/1 -> buscreator/5  "LocationZDefined"
  GND_LocationZ/1 -> buscreator/6  "LocationZ"
  GND_OrientationRollDefined/1 -> buscreator/7  "OrientationRollDefined"
  GND_OrientationRoll/1 -> buscreator/8  "OrientationRoll"
  GND_OrientationPitchDefined/1 -> buscreator/9  "OrientationPitchDefined"
  GND_OrientationPitch/1 -> buscreator/10  "OrientationPitch"
  GND_OrientationYawDefined/1 -> buscreator/11  "OrientationYawDefined"
  GND_OrientationYaw/1 -> buscreator/12  "OrientationYaw"
  GND_FovAzimuthDefined/1 -> buscreator/13  "FovAzimuthDefined"
  GND_FovAzimuth/1 -> buscreator/14  "FovAzimuth"
  GND_FovElevationDefined/1 -> buscreator/15  "FovElevationDefined"
  GND_FovElevation/1 -> buscreator/16  "FovElevation"
  GND_NearClippingDistanceDefined/1 -> buscreator/17  "NearClippingDistanceDefined"
  GND_NearClippingDistance/1 -> buscreator/18  "NearClippingDistance"
  GND_FarClippingDistanceDefined/1 -> buscreator/19  "FarClippingDistanceDefined"
  GND_FarClippingDistance/1 -> buscreator/20  "FarClippingDistance"
  buscreator/1 -> bus/1

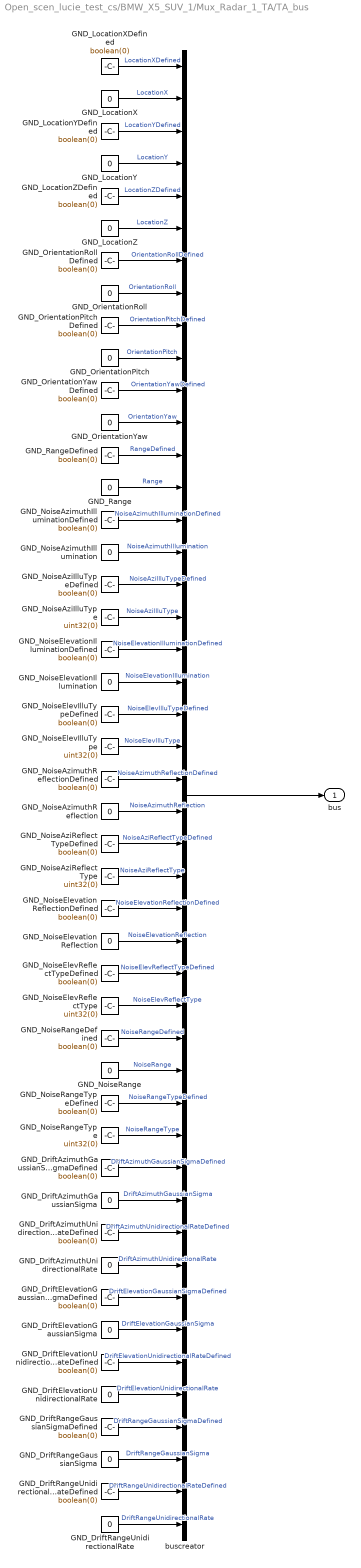
== system Open_scen_lucie_test_cs/BMW_X5_SUV_1/Mux_Radar_1_TA/TA_bus ==
  GND_DriftAzimuthGaussianSigma : Constant  Value=0
  GND_DriftAzimuthGaussianSigmaDefined : Constant  Value=boolean(0)
  GND_DriftAzimuthUnidirectionalRate : Constant  Value=0
  GND_DriftAzimuthUnidirectionalRateDefined : Constant  Value=boolean(0)
  GND_DriftElevationGaussianSigma : Constant  Value=0
  GND_DriftElevationGaussianSigmaDefined : Constant  Value=boolean(0)
  GND_DriftElevationUnidirectionalRate : Constant  Value=0
  GND_DriftElevationUnidirectionalRateDefined : Constant  Value=boolean(0)
  GND_DriftRangeGaussianSigma : Constant  Value=0
  GND_DriftRangeGaussianSigmaDefined : Constant  Value=boolean(0)
  GND_DriftRangeUnidirectionalRate : Constant  Value=0
  GND_DriftRangeUnidirectionalRateDefined : Constant  Value=boolean(0)
  GND_LocationX : Constant  Value=0
  GND_LocationXDefined : Constant  Value=boolean(0)
  GND_LocationY : Constant  Value=0
  GND_LocationYDefined : Constant  Value=boolean(0)
  GND_LocationZ : Constant  Value=0
  GND_LocationZDefined : Constant  Value=boolean(0)
  GND_NoiseAziIlluType : Constant  Value=uint32(0)
  GND_NoiseAziIlluTypeDefined : Constant  Value=boolean(0)
  GND_NoiseAziReflectType : Constant  Value=uint32(0)
  GND_NoiseAziReflectTypeDefined : Constant  Value=boolean(0)
  GND_NoiseAzimuthIllumination : Constant  Value=0
  GND_NoiseAzimuthIlluminationDefined : Constant  Value=boolean(0)
  GND_NoiseAzimuthReflection : Constant  Value=0
  GND_NoiseAzimuthReflectionDefined : Constant  Value=boolean(0)
  GND_NoiseElevIlluType : Constant  Value=uint32(0)
  GND_NoiseElevIlluTypeDefined : Constant  Value=boolean(0)
  GND_NoiseElevReflectType : Constant  Value=uint32(0)
  GND_NoiseElevReflectTypeDefined : Constant  Value=boolean(0)
  GND_NoiseElevationIllumination : Constant  Value=0
  GND_NoiseElevationIlluminationDefined : Constant  Value=boolean(0)
  GND_NoiseElevationReflection : Constant  Value=0
  GND_NoiseElevationReflectionDefined : Constant  Value=boolean(0)
  GND_NoiseRange : Constant  Value=0
  GND_NoiseRangeDefined : Constant  Value=boolean(0)
  GND_NoiseRangeType : Constant  Value=uint32(0)
  GND_NoiseRangeTypeDefined : Constant  Value=boolean(0)
  GND_OrientationPitch : Constant  Value=0
  GND_OrientationPitchDefined : Constant  Value=boolean(0)
  GND_OrientationRoll : Constant  Value=0
  GND_OrientationRollDefined : Constant  Value=boolean(0)
  GND_OrientationYaw : Constant  Value=0
  GND_OrientationYawDefined : Constant  Value=boolean(0)
  GND_Range : Constant  Value=0
  GND_RangeDefined : Constant  Value=boolean(0)
  buscreator : BusCreator  Inputs=46  OutDataTypeStr=Bus: PRESCAN_SCANNERSENSOR_TA  NonVirtualBus=on
  bus : Outport  OutDataTypeStr=Bus: PRESCAN_SCANNERSENSOR_TA
  wires:
  GND_LocationXDefined/1 -> buscreator/1  "LocationXDefined"
  GND_LocationX/1 -> buscreator/2  "LocationX"
  GND_LocationYDefined/1 -> buscreator/3  "LocationYDefined"
  GND_LocationY/1 -> buscreator/4  "LocationY"
  GND_LocationZDefined/1 -> buscreator/5  "LocationZDefined"
  GND_LocationZ/1 -> buscreator/6  "LocationZ"
  GND_OrientationRollDefined/1 -> buscreator/7  "OrientationRollDefined"
  GND_OrientationRoll/1 -> buscreator/8  "OrientationRoll"
  GND_OrientationPitchDefined/1 -> buscreator/9  "OrientationPitchDefined"
  GND_OrientationPitch/1 -> buscreator/10  "OrientationPitch"
  GND_OrientationYawDefined/1 -> buscreator/11  "OrientationYawDefined"
  GND_OrientationYaw/1 -> buscreator/12  "OrientationYaw"
  GND_RangeDefined/1 -> buscreator/13  "RangeDefined"
  GND_Range/1 -> buscreator/14  "Range"
  GND_NoiseAzimuthIlluminationDefined/1 -> buscreator/15  "NoiseAzimuthIlluminationDefined"
  GND_NoiseAzimuthIllumination/1 -> buscreator/16  "NoiseAzimuthIllumination"
  GND_NoiseAziIlluTypeDefined/1 -> buscreator/17  "NoiseAziIlluTypeDefined"
  GND_NoiseAziIlluType/1 -> buscreator/18  "NoiseAziIlluType"
  GND_NoiseElevationIlluminationDefined/1 -> buscreator/19  "NoiseElevationIlluminationDefined"
  GND_NoiseElevationIllumination/1 -> buscreator/20  "NoiseElevationIllumination"
  GND_NoiseElevIlluTypeDefined/1 -> buscreator/21  "NoiseElevIlluTypeDefined"
  GND_NoiseElevIlluType/1 -> buscreator/22  "NoiseElevIlluType"
  GND_NoiseAzimuthReflectionDefined/1 -> buscreator/23  "NoiseAzimuthReflectionDefined"
  GND_NoiseAzimuthReflection/1 -> buscreator/24  "NoiseAzimuthReflection"
  GND_NoiseAziReflectTypeDefined/1 -> buscreator/25  "NoiseAziReflectTypeDefined"
  GND_NoiseAziReflectType/1 -> buscreator/26  "NoiseAziReflectType"
  GND_NoiseElevationReflectionDefined/1 -> buscreator/27  "NoiseElevationReflectionDefined"
  GND_NoiseElevationReflection/1 -> buscreator/28  "NoiseElevationReflection"
  GND_NoiseElevReflectTypeDefined/1 -> buscreator/29  "NoiseElevReflectTypeDefined"
  GND_NoiseElevReflectType/1 -> buscreator/30  "NoiseElevReflectType"
  GND_NoiseRangeDefined/1 -> buscreator/31  "NoiseRangeDefined"
  GND_NoiseRange/1 -> buscreator/32  "NoiseRange"
  GND_NoiseRangeTypeDefined/1 -> buscreator/33  "NoiseRangeTypeDefined"
  GND_NoiseRangeType/1 -> buscreator/34  "NoiseRangeType"
  GND_DriftAzimuthGaussianSigmaDefined/1 -> buscreator/35  "DriftAzimuthGaussianSigmaDefined"
  GND_DriftAzimuthGaussianSigma/1 -> buscreator/36  "DriftAzimuthGaussianSigma"
  GND_DriftAzimuthUnidirectionalRateDefined/1 -> buscreator/37  "DriftAzimuthUnidirectionalRateDefined"
  GND_DriftAzimuthUnidirectionalRate/1 -> buscreator/38  "DriftAzimuthUnidirectionalRate"
  GND_DriftElevationGaussianSigmaDefined/1 -> buscreator/39  "DriftElevationGaussianSigmaDefined"
  GND_DriftElevationGaussianSigma/1 -> buscreator/40  "DriftElevationGaussianSigma"
  GND_DriftElevationUnidirectionalRateDefined/1 -> buscreator/41  "DriftElevationUnidirectionalRateDefined"
  GND_DriftElevationUnidirectionalRate/1 -> buscreator/42  "DriftElevationUnidirectionalRate"
  GND_DriftRangeGaussianSigmaDefined/1 -> buscreator/43  "DriftRangeGaussianSigmaDefined"
  GND_DriftRangeGaussianSigma/1 -> buscreator/44  "DriftRangeGaussianSigma"
  GND_DriftRangeUnidirectionalRateDefined/1 -> buscreator/45  "DriftRangeUnidirectionalRateDefined"
  GND_DriftRangeUnidirectionalRate/1 -> buscreator/46  "DriftRangeUnidirectionalRate"
  buscreator/1 -> bus/1

== system Open_scen_lucie_test_cs/BMW_X5_SUV_1/SELF_Demux/compas converter ==
  rotz [rad] : Inport
  cart2compas : Subsystem
  rad2deg : Gain  Gain=180/pi
  heading [deg] : Outport
  wires:
  rad2deg/1 -> cart2compas/1(Angle [deg])
  rotz [rad]/1 -> rad2deg/1
  cart2compas/1(heading [deg]) -> heading [deg]/1

== system Open_scen_lucie_test_cs/Male_200_1/Animation/animation mode ==
  vel : Inport
  Data Type Conversion : DataTypeConversion  OutDataTypeStr=int32
  Fcn : Fcn  Expr=u(1)^2+u(2)^2+u(3)^2
  Walking : simulink/Logic and Bit Operations/Compare To Zero  relop=~=  OutDataTypeStr=uint8  ZeroCross=off
  mode : Outport
  wires:
  Data Type Conversion/1 -> mode/1
  Walking/1 -> Data Type Conversion/1
  Fcn/1 -> Walking/1
  vel/1 -> Fcn/1

== system Open_scen_lucie_test_cs/Male_200_1/Animation/elapsed track ==
  vel : Inport
  Discrete-Time Integrator : DiscreteIntegrator  SampleTime=-1  ICPrevOutput=DiscIntNeverNeededParam  ICPrevScaledInput=DiscIntNeverNeededParam
  Fcn : Fcn  Expr=sqrt(u(1)^2 + u(2)^2 + u(3)^2)
  s : Outport
  wires:
  Discrete-Time Integrator/1 -> s/1
  vel/1 -> Fcn/1
  Fcn/1 -> Discrete-Time Integrator/1

== system Open_scen_lucie_test_cs/Male_200_1/Dynamics_Empty/MuxState ==
  note: mode: Dynamics
  note: mode: Positioning
  note: mode: Dynamics
      | VelVEHICLE
      | wrt VEH
  note: AnglesVEHICLE
      | wrtGLOB
  note: For state mode 'Dynamic' positions
      | are not taken into account, as they
      | are computed by integrating velocity.
      | Click annotation for Help.
  x [m] : Inport  SampleTime=TimeStep
  y [m] : Inport  Port=2  SampleTime=TimeStep
  z [m] : Inport  Port=3  SampleTime=TimeStep
  dx [m/s] : Inport  Port=4  SampleTime=TimeStep
  dy [m/s] : Inport  Port=5  SampleTime=TimeStep
  dz [m/s] : Inport  Port=6  SampleTime=TimeStep
  R [rad] : Inport  Port=7  SampleTime=TimeStep
  P [rad] : Inport  Port=8  SampleTime=TimeStep
  Y [rad] : Inport  Port=9  SampleTime=TimeStep
  Constant : Constant  DisableCoverage=on  Value=positioningmode
  Discrete-Time Integrator : DiscreteIntegrator  SampleTime=TimeStep  ICPrevOutput=DiscIntNeverNeededParam  ICPrevScaledInput=DiscIntNeverNeededParam
  Ground : Ground
  Ground1 : Ground
  Mux1 : Mux  Inputs=[3 3]
  Mux2 : Mux  Inputs=3
  Mux3 : Mux  Inputs=3
  Mux4 : Mux  Inputs=3
  Mux5 : Mux  Inputs=[3 3]
  Mux6 : Mux  Inputs=[6 3]
  Switch : Switch  Threshold=0.5
  Transformation_BODY2GLOBAL : PreScanSimulinkLibrary/Simple_Vehicle_Dynamics/Chassis/MuxDynState/Transformation_BODY2GLOBAL  SystemSampleTime=-1
  mux3 : Mux  Inputs=3
  state : Outport
  wires:
  Constant/1 -> Switch/2
  Mux6/1 -> state/1
  Mux4/1 -> Mux1/1
  Mux5/1 -> Switch/3
  Mux1/1 -> Switch/1
  Switch/1 -> Mux6/1  "PosVeh wrt  GLOB"
  P [rad]/1 -> Mux3/2
  R [rad]/1 -> Mux3/1
  dz [m/s]/1 -> Mux2/3
  dy [m/s]/1 -> Mux2/2
  dx [m/s]/1 -> Mux2/1
  z [m]/1 -> Mux4/3
  y [m]/1 -> Mux4/2
  x [m]/1 -> Mux4/1
  Ground1/1 -> mux3/2  "pitch"
  Y [rad]/1 -> mux3/3, Mux3/3  "yaw"
  Mux3/1 -> Mux6/2
  Transformation_BODY2GLOBAL/1 -> Discrete-Time Integrator/1, Mux5/2  "VelVEH wrt  GLOB"
  mux3/1 -> Transformation_BODY2GLOBAL/2
  Ground/1 -> mux3/1  "roll"
  Mux2/1 -> Mux1/2, Transformation_BODY2GLOBAL/1
  Discrete-Time Integrator/1 -> Mux5/1  "PosVEH wrt  GLOB"
